simulink model "Grid_Forming_Converters_Microgrid_Github"  (R2020b)
settings: Solver=VariableStepAuto  StartTime=0.0  StopTime=1  RelTol=1e-3
values from neighbouring files (symbols this model uses):
  C_fi_1DG = 50*10^-6    (= 5e-05)    [Script_Primary_Secondary_Controller_GITHUB.m]
  C_fi_2DG = 50*10^-6    (= 5e-05)    [Script_Primary_Secondary_Controller_GITHUB.m]
  C_fi_3DG = 50*10^-6    (= 5e-05)    [Script_Primary_Secondary_Controller_GITHUB.m]
  C_fi_4DG = 50*10^-6    (= 5e-05)    [Script_Primary_Secondary_Controller_GITHUB.m]
  Kff_i_1DG = 0.75    [Script_Primary_Secondary_Controller_GITHUB.m]
  Kff_i_2DG = 0.75    [Script_Primary_Secondary_Controller_GITHUB.m]
  Kff_i_3DG = 0.75    [Script_Primary_Secondary_Controller_GITHUB.m]
  Kff_i_4DG = 0.75    [Script_Primary_Secondary_Controller_GITHUB.m]
  ki = 142500    [Script_Primary_Secondary_Controller_GITHUB.m]
  Kii_1DG = 20000    [Script_Primary_Secondary_Controller_GITHUB.m]
  Kii_2DG = 20000    [Script_Primary_Secondary_Controller_GITHUB.m]
  Kii_3DG = 16000    [Script_Primary_Secondary_Controller_GITHUB.m]
  Kii_4DG = 16000    [Script_Primary_Secondary_Controller_GITHUB.m]
  Kiv_1DG = 420    [Script_Primary_Secondary_Controller_GITHUB.m]
  Kiv_2DG = 420    [Script_Primary_Secondary_Controller_GITHUB.m]
  Kiv_3DG = 390    [Script_Primary_Secondary_Controller_GITHUB.m]
  Kiv_4DG = 390    [Script_Primary_Secondary_Controller_GITHUB.m]
  kp = 285    [Script_Primary_Secondary_Controller_GITHUB.m]
  Kpi_1DG = 15    [Script_Primary_Secondary_Controller_GITHUB.m]
  Kpi_2DG = 15    [Script_Primary_Secondary_Controller_GITHUB.m]
  Kpi_3DG = 10.5    [Script_Primary_Secondary_Controller_GITHUB.m]
  Kpi_4DG = 10.5    [Script_Primary_Secondary_Controller_GITHUB.m]
  Kpv_1DG = 0.1    [Script_Primary_Secondary_Controller_GITHUB.m]
  Kpv_2DG = 0.1    [Script_Primary_Secondary_Controller_GITHUB.m]
  Kpv_3DG = 0.05    [Script_Primary_Secondary_Controller_GITHUB.m]
  Kpv_4DG = 0.05    [Script_Primary_Secondary_Controller_GITHUB.m]
  L_ci_1DG = 0.35*10^-3    (= 0.00035)    [Script_Primary_Secondary_Controller_GITHUB.m]
  L_ci_2DG = 0.35*10^-3    (= 0.00035)    [Script_Primary_Secondary_Controller_GITHUB.m]
  L_fi_1DG = 1.35*10^-3    (= 0.00135)    [Script_Primary_Secondary_Controller_GITHUB.m]
  L_fi_2DG = 1.35*10^-3    (= 0.00135)    [Script_Primary_Secondary_Controller_GITHUB.m]
  L_fi_3DG = 1.35*10^-3    (= 0.00135)    [Script_Primary_Secondary_Controller_GITHUB.m]
  L_fi_4DG = 1.35*10^-3    (= 0.00135)    [Script_Primary_Secondary_Controller_GITHUB.m]
  L_line_1 = 318*10^-6    (= 0.000318)    [Script_Primary_Secondary_Controller_GITHUB.m]
  L_line_2 = 1847*10^-6    (= 0.001847)    [Script_Primary_Secondary_Controller_GITHUB.m]
  L_line_3 = 318*10^-6    (= 0.000318)    [Script_Primary_Secondary_Controller_GITHUB.m]
  L_load_1 = (X_load_1)/(2*pi*f)    (= 0.0477464829276)    [Script_Primary_Secondary_Controller_GITHUB.m]
  L_load_2 = (X_load_2)/(2*pi*f)    (= 0.0318309886184)    [Script_Primary_Secondary_Controller_GITHUB.m]
  L_load_3 = (X_load_3)/(2*pi*f)    (= 0.0318309886184)    [Script_Primary_Secondary_Controller_GITHUB.m]
  L_load_4 = (X_load_4)/(2*pi*f)    (= 0.0477464829276)    [Script_Primary_Secondary_Controller_GITHUB.m]
  m_P_1DG = 9.4*10^-5    (= 9.4e-05)    [Script_Primary_Secondary_Controller_GITHUB.m]
  m_P_2DG = 9.4*10^-5    (= 9.4e-05)    [Script_Primary_Secondary_Controller_GITHUB.m]
  m_P_3DG = 12.5*10^-5    (= 0.000125)    [Script_Primary_Secondary_Controller_GITHUB.m]
  m_P_4DG = 12.5*10^-5    (= 0.000125)    [Script_Primary_Secondary_Controller_GITHUB.m]
  n_Q_1DG = 1.3*10^-3    (= 0.0013)    [Script_Primary_Secondary_Controller_GITHUB.m]
  n_Q_2DG = 1.3*10^-3    (= 0.0013)    [Script_Primary_Secondary_Controller_GITHUB.m]
  n_Q_3DG = 1.5*10^-3    (= 0.0015)    [Script_Primary_Secondary_Controller_GITHUB.m]
  n_Q_4DG = 1.5*10^-3    (= 0.0015)    [Script_Primary_Secondary_Controller_GITHUB.m]
  R_ci_1DG = 0.03    [Script_Primary_Secondary_Controller_GITHUB.m]
  R_ci_2DG = 0.03    [Script_Primary_Secondary_Controller_GITHUB.m]
  R_fi_1DG = 0.1    [Script_Primary_Secondary_Controller_GITHUB.m]
  R_fi_2DG = 0.1    [Script_Primary_Secondary_Controller_GITHUB.m]
  R_fi_3DG = 0.1    [Script_Primary_Secondary_Controller_GITHUB.m]
  R_line_1 = 0.23    [Script_Primary_Secondary_Controller_GITHUB.m]
  R_line_2 = 0.35    [Script_Primary_Secondary_Controller_GITHUB.m]
  R_line_3 = 0.23    [Script_Primary_Secondary_Controller_GITHUB.m]
  R_load_1 = 30    [Script_Primary_Secondary_Controller_GITHUB.m]
  R_load_2 = 20    [Script_Primary_Secondary_Controller_GITHUB.m]
  R_load_3 = 25    [Script_Primary_Secondary_Controller_GITHUB.m]
  R_load_4 = 25    [Script_Primary_Secondary_Controller_GITHUB.m]
  Ts_1DG = 2e-6    (= 2e-06)    [Script_Primary_Secondary_Controller_GITHUB.m]
  w_base_1DG = 2*pi*f_1DG    (= 314.159265359)    [Script_Primary_Secondary_Controller_GITHUB.m]
  w_base_2DG = 2*pi*f_2DG    (= 314.159265359)    [Script_Primary_Secondary_Controller_GITHUB.m]
  w_base_3DG = 2*pi*f_3DG    (= 314.159265359)    [Script_Primary_Secondary_Controller_GITHUB.m]
  w_base_4DG = 2*pi*f_4DG    (= 314.159265359)    [Script_Primary_Secondary_Controller_GITHUB.m]
  wci_1DG = 31.41    [Script_Primary_Secondary_Controller_GITHUB.m]
  wci_2DG = 31.41    [Script_Primary_Secondary_Controller_GITHUB.m]
  wci_3DG = 31.41    [Script_Primary_Secondary_Controller_GITHUB.m]
  wci_4DG = 31.41    [Script_Primary_Secondary_Controller_GITHUB.m]
undefined symbols (not defined in the file or in its folder): L_i_1DG
libraries: powerlib x140, powerlib_meascontrol x68, pid_lib x20
(part 2 of 6)

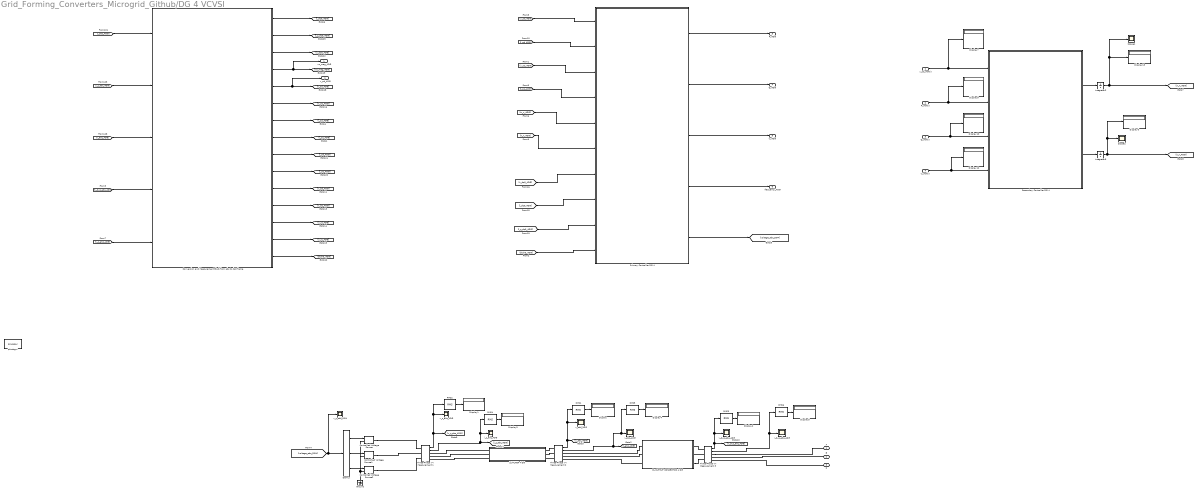
== system Grid_Forming_Converters_Microgrid_Github/DG 4 VCVSI  ==
  v_od_matrix : Inport
  P_matrix : Inport  Port=2
  Q_matrix : Inport  Port=3
  w_matrix : Inport  Port=4
  Controlled Voltage Source : powerlib/Electrical Sources/Controlled Voltage Source  Initialize=on  Source_Type=AC  Amplitude=0  Phase=0  Frequency=0  Measurements=None
  Controlled Voltage Source1 : powerlib/Electrical Sources/Controlled Voltage Source  Initialize=on  Source_Type=AC  Amplitude=0  Phase=0  Frequency=0  Measurements=None
  Controlled Voltage Source2 : powerlib/Electrical Sources/Controlled Voltage Source  Initialize=on  Source_Type=AC  Amplitude=0  Phase=0  Frequency=0  Measurements=None
  Conversion and Measurement Block from abc to dq0 frame : Subsystem
  Demux : Demux  Outputs=3
  Display{,1..7,9..10,12..13} (12 alike) : Display
  Ground : powerlib/Elements/Ground  LConnTagsString=a
  Integrator2 : Integrator
  Integrator3 : Integrator
  LC FILTER 4 DG : Subsystem
  Primary Controller DG 4 : Subsystem
  RL OUTPUT CONNECTOR 4 DG : Subsystem
  RMS{1..3,5..6} (5 alike) : powerlib_meascontrol/Measurements/RMS  TrueRMS=off  Freq=50  RMSInit=1  Ts=Ts_1DG
  RMS4 : powerlib_meascontrol/Measurements/RMS  TrueRMS=on  Freq=50  RMSInit=1  Ts=Ts_1DG
  Scope1 : Scope
  Scope2 : Scope
  Secondary Controller DG 4 : MATLAB Function  TreatAsAtomicUnit=on
  Three-Phase V-I Measurement 1 : powerlib/Measurements/Three-Phase V-I Measurement  VoltageMeasurement=phase-to-phase  SetLabelV=off  LabelV=Vabc  Vpu=off  VpuLL=off  CurrentMeasurement=yes  SetLabelI=off  LabelI=Iabc  Ipu=off  Pbase=45000  Vbase=380  OutputType=Complex  PhasorSimulation=off  PSBequivalent=0
  Three-Phase V-I Measurement 2 : powerlib/Measurements/Three-Phase V-I Measurement  VoltageMeasurement=phase-to-phase  SetLabelV=off  LabelV=Vabc  Vpu=off  VpuLL=off  CurrentMeasurement=yes  SetLabelI=off  LabelI=Iabc  Ipu=off  Pbase=45000  Vbase=380  OutputType=Complex  PhasorSimulation=off  PSBequivalent=0
  Three-Phase V-I Measurement 3 : powerlib/Measurements/Three-Phase V-I Measurement  VoltageMeasurement=phase-to-phase  SetLabelV=off  LabelV=Vabc  Vpu=off  VpuLL=off  CurrentMeasurement=yes  SetLabelI=off  LabelI=Iabc  Ipu=off  Pbase=45000  Vbase=380  OutputType=Complex  PhasorSimulation=off  PSBequivalent=0
  i_abc_4DG : Scope
  i_bus_abc_4DG : Scope
  i_s_abc_4DG : Scope
  powergui : powerlib/powergui  Priority=1  SimulationMode=Discrete  SampleTime=2e-6  frequency=60  Iterations=50  frequencyindice=0  Pbase=100e6  ErrMax=1e-4  UnitsV=kV  UnitsW=MW  buscounter=0  FunctionMessages=off  echomessages=off  EnableUseOfTLC=off  CurrentSourceSwitches=off  DisableSnubberDevices=off  DisableRonSwitches=off  DisableVfSwitches=off  DisplayEquations=off  AutomaticDiscreteSolvers=off  SolverType=Tustin/Backward Euler (TBE)  Interpol=off  ExternalGateDelay=off  methode=off  Ts=100  x0status=blocks  SPID=on  SwTol=0  HookPort=off  NonlinearTolerance=1e-4  nMaxIteration=100  ContinueOnMaxIteration=off  RestoreLinks=warning  ResistiveCurrentMeasurement=off  Frange=[0:2:500]  Ylog=off  Xlog=on  ShowGrid=off  save=off  variable=ZData  structure=0  ZoomFFT=off  StartTime=0.0  cycles=1  DisplayStyle=1  fundamental=60  FreqAxis=off  MaxFrequency=1000  frequencyindicesteady=1  RmsSteady=1  display=off
  v_abc_4DG : Scope
  v_bus_abc_4DG : Scope
  v_s_abc_4DG : Scope
  v_s_abc_DG4 : Scope
  A : PMIOPort  Side=Right
  B : PMIOPort  Port=2  Side=Right
  C : PMIOPort  Port=3  Side=Right
  vo_mag_4DG : Outport
  v_od_4DG : Outport  Port=2
  P_4DG : Outport  Port=3
  Q_4DG : Outport  Port=4
  w_4DG : Outport  Port=5
  frequency_4DG : Outport  Port=6
  wires:
  Three-Phase V-I Measurement 2/1 -> RMS1/1, v_abc_4DG/1, [v_abc_4DG]
  Three-Phase V-I Measurement 1/1 -> [v_s_abc_4DG], RMS2/1, v_s_abc_4DG/1
  Three-Phase V-I Measurement 1/2 -> RMS4/1, i_s_abc_4DG/1, [i_s_abc_4DG]
  RMS3/1 -> Display2/1
  Three-Phase V-I Measurement 3/1 -> [v_bus_abc_4DG], RMS3/1, v_bus_abc_4DG/1
  RMS5/1 -> Display4/1
  Three-Phase V-I Measurement 2/2 -> RMS5/1, i_abc_4DG/1, [i_abc_4DG]
  RMS1/1 -> Display/1
  Three-Phase V-I Measurement 3/2 -> RMS6/1, i_bus_abc_4DG/1
  RMS6/1 -> Display5/1
  RMS2/1 -> Display1/1
  RMS4/1 -> Display3/1
  Primary Controller DG 4/1(P_4DG) -> P_4DG/1
  Primary Controller DG 4/5(voltage_abc_DG4) -> [voltage_abc_DG4]
  [V_n_4DG] -> Primary Controller DG 4/6(V_n_4DG)
  Primary Controller DG 4/4(frequency_4DG) -> frequency_4DG/1
  [w_n_4DG] -> Primary Controller DG 4/5(w_n_4DG)
  [voltage_abc_DG4] -> Demux/1, v_s_abc_DG4/1
  Demux/1 -> Controlled Voltage Source/1
  Demux/2 -> Controlled Voltage Source1/1
  Demux/3 -> Controlled Voltage Source2/1
  [i_abc_4DG] -> Conversion and Measurement Block from abc to dq0 frame/1(i_abc_4DG)
  [i_s_abc_4DG] -> Conversion and Measurement Block from abc to dq0 frame/2(i_s_abc_4DG)
  [v_abc_4DG] -> Conversion and Measurement Block from abc to dq0 frame/3(v_abc_4DG)
  Conversion and Measurement Block from abc to dq0 frame/8(i_1q_4DG) -> [i_1q_4DG]
  Conversion and Measurement Block from abc to dq0 frame/7(i_1d_4DG) -> [i_1d_4DG]
  Conversion and Measurement Block from abc to dq0 frame/6(v_oq_4DG) -> [v_oq_4DG]
  Conversion and Measurement Block from abc to dq0 frame/4(vo_mag_4DG) -> [vo_mag_4DG], vo_mag_4DG/1
  Conversion and Measurement Block from abc to dq0 frame/5(v_od_4DG) -> [v_od_4DG], v_od_4DG/1
  [i_oq_4DG] -> Primary Controller DG 4/4(i_oq_4DG)
  [v_od_4DG] -> Primary Controller DG 4/1(v_od_4DG)
  [v_oq_4DG] -> Primary Controller DG 4/3(v_oq_4DG)
  [i_od_4DG] -> Primary Controller DG 4/2(i_od_4DG)
  [i_dq0_4DG] -> Primary Controller DG 4/8(i_dq0_4DG)
  [v_dq0_4DG] -> Primary Controller DG 4/7(v_dq0_4DG)
  [i_s_dq0_4DG] -> Primary Controller DG 4/9(i_s_dq0_4DG)
  Conversion and Measurement Block from abc to dq0 frame/9(i_od_4DG) -> [i_od_4DG]
  Conversion and Measurement Block from abc to dq0 frame/10(i_oq_4DG) -> [i_oq_4DG]
  Conversion and Measurement Block from abc to dq0 frame/15(alpha_4DG) -> [alpha_4DG]
  Conversion and Measurement Block from abc to dq0 frame/1(i_dq0_4DG) -> [i_dq0_4DG]
  Conversion and Measurement Block from abc to dq0 frame/2(i_s_dq0_4DG) -> [i_s_dq0_4DG]
  Conversion and Measurement Block from abc to dq0 frame/3(v_dq0_4DG) -> [v_dq0_4DG]
  [alpha_4DG] -> Primary Controller DG 4/10(alpha_4DG)
  Primary Controller DG 4/3(w_4DG) -> w_4DG/1
  Primary Controller DG 4/2(Q_4DG) -> Q_4DG/1
  [v_bus_abc_4DG] -> Conversion and Measurement Block from abc to dq0 frame/4(v_bus_abc_4DG)
  [v_s_abc_4DG] -> Conversion and Measurement Block from abc to dq0 frame/5(v_s_abc_4DG)
  Conversion and Measurement Block from abc to dq0 frame/11(v_bd_4DG) -> [v_bd_4DG]
  Conversion and Measurement Block from abc to dq0 frame/12(v_bq_4DG) -> [v_bq_4DG]
  Conversion and Measurement Block from abc to dq0 frame/14(v_iq_4DG) -> [v_iq_4DG]
  Conversion and Measurement Block from abc to dq0 frame/13(v_id_4DG) -> [v_id_4DG]
  Integrator3/1 -> [V_n_4DG], Display6/1, Scope2/1
  Secondary Controller DG 4/1(v_f_4DG) -> Integrator2/1
  Integrator2/1 -> [w_n_4DG], Scope1/1, Display13/1
  Secondary Controller DG 4/2(v_v_4DG) -> Integrator3/1
  v_od_matrix/1 -> Display7/1, Secondary Controller DG 4/1(v_od_matrix)
  P_matrix/1 -> Display9/1, Secondary Controller DG 4/2(P_matrix)
  Q_matrix/1 -> Display10/1, Secondary Controller DG 4/3(Q_matrix)
  w_matrix/1 -> Display12/1, Secondary Controller DG 4/4(w_matrix)
  connections:
  RL OUTPUT CONNECTOR 4 DG/LConn2 -- Three-Phase V-I Measurement 2/RConn2
  LC FILTER 4 DG/LConn2 -- Three-Phase V-I Measurement 1/RConn2
  RL OUTPUT CONNECTOR 4 DG/LConn1 -- Three-Phase V-I Measurement 2/RConn1
  C/RConn1 -- Three-Phase V-I Measurement 3/RConn3
  Three-Phase V-I Measurement 2/LConn3 -- LC FILTER 4 DG/RConn3
  Three-Phase V-I Measurement 3/RConn1 -- A/RConn1
  B/RConn1 -- Three-Phase V-I Measurement 3/RConn2
  Controlled Voltage Source1/RConn1 -- Three-Phase V-I Measurement 1/LConn2
  RL OUTPUT CONNECTOR 4 DG/LConn3 -- Three-Phase V-I Measurement 2/RConn3
  Three-Phase V-I Measurement 3/LConn1 -- RL OUTPUT CONNECTOR 4 DG/RConn1
  Three-Phase V-I Measurement 2/LConn1 -- LC FILTER 4 DG/RConn1
  Three-Phase V-I Measurement 3/LConn2 -- RL OUTPUT CONNECTOR 4 DG/RConn2
  RL OUTPUT CONNECTOR 4 DG/RConn3 -- Three-Phase V-I Measurement 3/LConn3
  Controlled Voltage Source2/RConn1 -- Three-Phase V-I Measurement 1/LConn3
  LC FILTER 4 DG/LConn3 -- Three-Phase V-I Measurement 1/RConn3
  LC FILTER 4 DG/LConn1 -- Three-Phase V-I Measurement 1/RConn1
  Three-Phase V-I Measurement 2/LConn2 -- LC FILTER 4 DG/RConn2
  Controlled Voltage Source/RConn1 -- Three-Phase V-I Measurement 1/LConn1
  Ground/LConn1 -- Controlled Voltage Source/LConn1 -- Controlled Voltage Source1/LConn1 -- Controlled Voltage Source2/LConn1

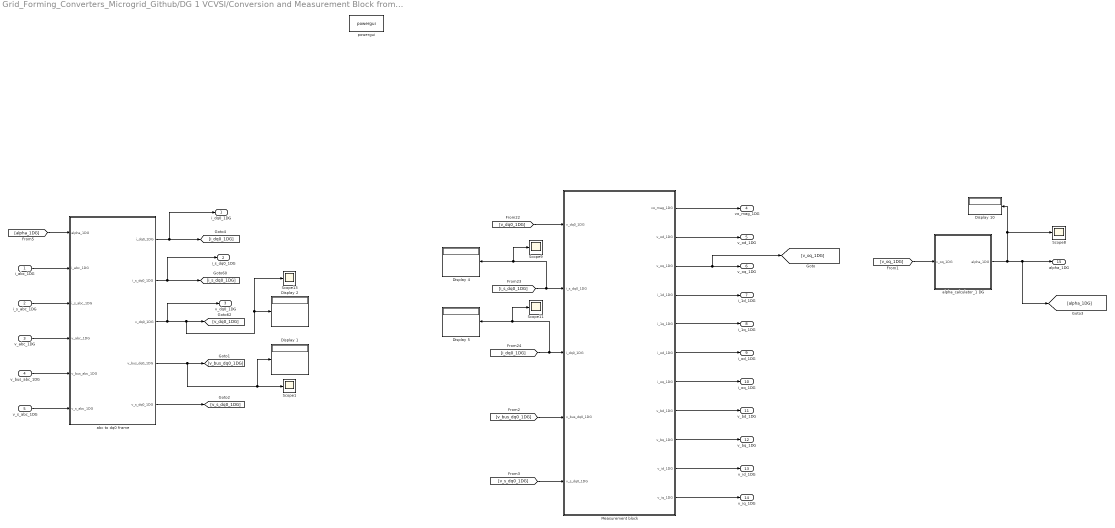
== system Grid_Forming_Converters_Microgrid_Github/DG 1 VCVSI/Conversion and Measurement Block from abc to dq0 frame ==
  i_abc_1DG : Inport
  i_s_abc_1DG : Inport  Port=2
  v_abc_1DG : Inport  Port=3
  v_bus_abc_1DG : Inport  Port=4
  v_s_abc_1DG : Inport  Port=5
  Display {1..2,4..5,10} (5 alike) : Display
      settings: Format=bank
  Measurement block : Subsystem
  Scope{1,8..9,11,13} (5 alike) : Scope
  abc to dq0 frame : Subsystem
  alpha_calculator_1 DG : Subsystem
  powergui : powerlib/powergui  Priority=1  SimulationMode=Discrete  SampleTime=2e-6  frequency=60  Iterations=50  frequencyindice=0  Pbase=100e6  ErrMax=1e-4  UnitsV=kV  UnitsW=MW  buscounter=0  FunctionMessages=off  echomessages=off  EnableUseOfTLC=off  CurrentSourceSwitches=off  DisableSnubberDevices=off  DisableRonSwitches=off  DisableVfSwitches=off  DisplayEquations=off  AutomaticDiscreteSolvers=off  SolverType=Tustin/Backward Euler (TBE)  Interpol=off  ExternalGateDelay=off  methode=off  Ts=100  x0status=blocks  SPID=on  SwTol=0  HookPort=off  NonlinearTolerance=1e-4  nMaxIteration=100  ContinueOnMaxIteration=off  RestoreLinks=warning  ResistiveCurrentMeasurement=off  Frange=[0:2:500]  Ylog=off  Xlog=on  ShowGrid=off  save=off  variable=ZData  structure=0  ZoomFFT=off  StartTime=0.0  cycles=1  DisplayStyle=1  fundamental=60  FreqAxis=off  MaxFrequency=1000  frequencyindicesteady=1  RmsSteady=1  display=off
  i_dq0_1DG : Outport
  i_s_dq0_1DG : Outport  Port=2
  v_dq0_1DG : Outport  Port=3
  vo_mag_1DG : Outport  Port=4
  v_od_1DG : Outport  Port=5
  v_oq_1DG : Outport  Port=6
  i_1d_1DG : Outport  Port=7
  i_1q_1DG : Outport  Port=8
  i_od_1DG : Outport  Port=9
  i_oq_1DG : Outport  Port=10
  v_bd_1DG : Outport  Port=11
  v_bq_1DG : Outport  Port=12
  v_id_1DG : Outport  Port=13
  v_iq_1DG : Outport  Port=14
  alpha_1DG : Outport  Port=15
  wires:
  Measurement block/5(i_1q_1DG) -> i_1q_1DG/1
  [i_dq0_1DG] -> Scope11/1, Display 5/1, Measurement block/3(i_dq0_1DG)
  abc to dq0 frame/2(i_s_dq0_1DG) -> i_s_dq0_1DG/1, [i_s_dq0_1DG]
  i_s_abc_1DG/1 -> abc to dq0 frame/3(i_s_abc_1DG)
  abc to dq0 frame/1(i_dq0_1DG) -> i_dq0_1DG/1, [i_dq0_1DG]
  Measurement block/4(i_1d_1DG) -> i_1d_1DG/1
  Measurement block/6(i_od_1DG) -> i_od_1DG/1
  abc to dq0 frame/3(v_dq0_1DG) -> v_dq0_1DG/1, Scope13/1, Display 2/1, [v_dq0_1DG]
  [v_dq0_1DG] -> Measurement block/1(v_dq0_1DG)
  i_abc_1DG/1 -> abc to dq0 frame/2(i_abc_1DG)
  Measurement block/2(v_od_1DG) -> v_od_1DG/1
  Measurement block/3(v_oq_1DG) -> [v_oq_1DG], v_oq_1DG/1
  v_abc_1DG/1 -> abc to dq0 frame/4(v_abc_1DG)
  Measurement block/7(i_oq_1DG) -> i_oq_1DG/1
  alpha_calculator_1 DG/1(alpha_1DG) -> [alpha_1DG], alpha_1DG/1, Display 10/1, Scope8/1
  [v_oq_1DG] -> alpha_calculator_1 DG/1(v_oq_1DG)
  [alpha_1DG] -> abc to dq0 frame/1(alpha_1DG)
  Measurement block/1(vo_mag_1DG) -> vo_mag_1DG/1
  [i_s_dq0_1DG] -> Scope9/1, Display 4/1, Measurement block/2(i_s_dq0_1DG)
  abc to dq0 frame/4(v_bus_dq0_1DG) -> [v_bus_dq0_1DG], Scope1/1, Display 1/1
  v_bus_abc_1DG/1 -> abc to dq0 frame/5(v_bus_abc_1DG)
  [v_bus_dq0_1DG] -> Measurement block/4(v_bus_dq0_1DG)
  Measurement block/8(v_bd_1DG) -> v_bd_1DG/1
  Measurement block/9(v_bq_1DG) -> v_bq_1DG/1
  v_s_abc_1DG/1 -> abc to dq0 frame/6(v_s_abc_1DG)
  abc to dq0 frame/5(v_s_dq0_1DG) -> [v_s_dq0_1DG]
  [v_s_dq0_1DG] -> Measurement block/5(v_s_dq0_1DG)
  Measurement block/10(v_id_1DG) -> v_id_1DG/1
  Measurement block/11(v_iq_1DG) -> v_iq_1DG/1

== system Grid_Forming_Converters_Microgrid_Github/DG 1 VCVSI/LC FILTER 1 DG ==
  C_a : powerlib/Elements/Series RLC Branch  LConnTagsString=__new0  RConnTagsString=__new0  BranchType=C  Resistance=1  Inductance=1e-3  SetiL0=off  InitialCurrent=0  Capacitance=C_fi_1DG  Setx0=off  InitialVoltage=165  Measurements=None
  C_b : powerlib/Elements/Series RLC Branch  LConnTagsString=__new0  RConnTagsString=__new0  BranchType=C  Resistance=1  Inductance=1e-3  SetiL0=off  InitialCurrent=0  Capacitance=C_fi_1DG  Setx0=off  InitialVoltage=165  Measurements=None
  C_c1 : powerlib/Elements/Series RLC Branch  LConnTagsString=__new0  RConnTagsString=__new0  BranchType=C  Resistance=1  Inductance=1e-3  SetiL0=off  InitialCurrent=0  Capacitance=C_fi_1DG  Setx0=off  InitialVoltage=165  Measurements=None
  Ground2 : powerlib/Elements/Ground  LConnTagsString=a
  Series RLC Branch : powerlib/Elements/Series RLC Branch  LConnTagsString=__new0  RConnTagsString=__new0  BranchType=L  Resistance=1  Inductance=L_fi_1DG  SetiL0=off  InitialCurrent=0  Capacitance=1e-6  Setx0=off  InitialVoltage=0  Measurements=None
  Series RLC Branch1 : powerlib/Elements/Series RLC Branch  LConnTagsString=__new0  RConnTagsString=__new0  BranchType=R  Resistance=R_fi_1DG  Inductance=L_i_1DG  SetiL0=off  InitialCurrent=0  Capacitance=1e-6  Setx0=off  InitialVoltage=0  Measurements=None
  Series RLC Branch2 : powerlib/Elements/Series RLC Branch  LConnTagsString=__new0  RConnTagsString=__new0  BranchType=R  Resistance=R_fi_1DG  Inductance=L_i_1DG  SetiL0=off  InitialCurrent=0  Capacitance=1e-6  Setx0=off  InitialVoltage=0  Measurements=None
  Series RLC Branch3 : powerlib/Elements/Series RLC Branch  LConnTagsString=__new0  RConnTagsString=__new0  BranchType=L  Resistance=1  Inductance=L_fi_1DG  SetiL0=off  InitialCurrent=0  Capacitance=1e-6  Setx0=off  InitialVoltage=0  Measurements=None
  Series RLC Branch4 : powerlib/Elements/Series RLC Branch  LConnTagsString=__new0  RConnTagsString=__new0  BranchType=R  Resistance=R_fi_1DG  Inductance=R_fi_1DG  SetiL0=off  InitialCurrent=0  Capacitance=1e-6  Setx0=off  InitialVoltage=0  Measurements=None
  Series RLC Branch5 : powerlib/Elements/Series RLC Branch  LConnTagsString=__new0  RConnTagsString=__new0  BranchType=L  Resistance=1  Inductance=L_fi_1DG  SetiL0=off  InitialCurrent=0  Capacitance=1e-6  Setx0=off  InitialVoltage=0  Measurements=None
  Series RLC Branch6 : PMIOPort  Side=Left
  Series RLC Branch7 : PMIOPort  Port=2  Side=Right
  Series RLC Branch8 : PMIOPort  Port=3  Side=Left
  Series RLC Branch9 : PMIOPort  Port=4  Side=Right
  Series RLC Branch10 : PMIOPort  Port=5  Side=Left
  Series RLC Branch11 : PMIOPort  Port=6  Side=Right
  connections:
  Series RLC Branch7/RConn1 -- C_c1/LConn1 -- Series RLC Branch/RConn1
  Series RLC Branch8/RConn1 -- Series RLC Branch2/LConn1
  Series RLC Branch6/RConn1 -- Series RLC Branch1/LConn1
  Series RLC Branch9/RConn1 -- C_b/LConn1 -- Series RLC Branch3/RConn1
  Series RLC Branch11/RConn1 -- C_a/LConn1 -- Series RLC Branch5/RConn1
  Series RLC Branch10/RConn1 -- Series RLC Branch4/LConn1
  C_b/RConn1 -- C_c1/RConn1 -- Ground2/LConn1 -- C_a/RConn1
  Series RLC Branch/LConn1 -- Series RLC Branch1/RConn1
  Series RLC Branch3/LConn1 -- Series RLC Branch2/RConn1
  Series RLC Branch4/RConn1 -- Series RLC Branch5/LConn1

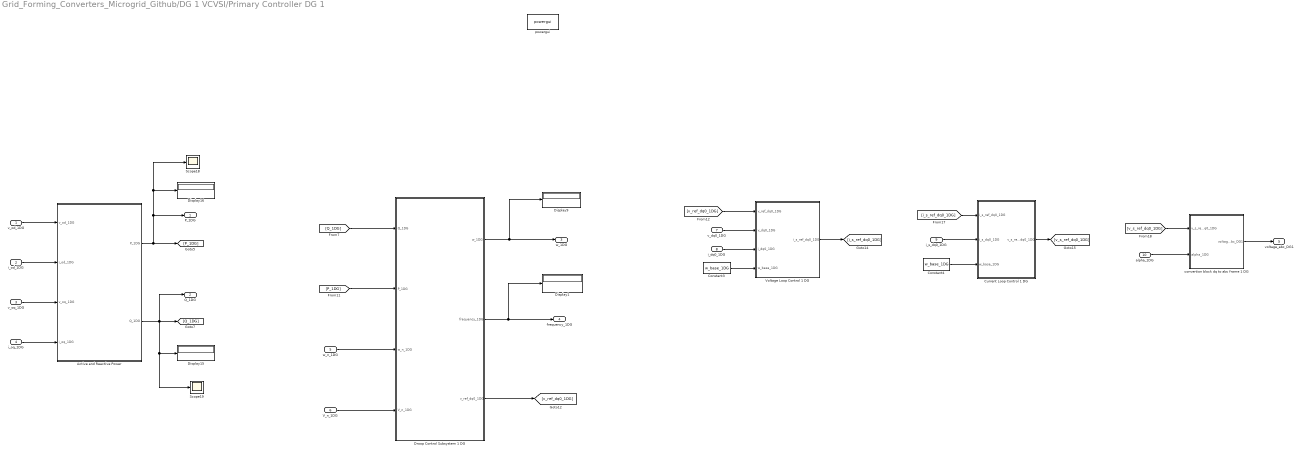
== system Grid_Forming_Converters_Microgrid_Github/DG 1 VCVSI/Primary Controller DG 1 ==
  v_od_1DG : Inport
  i_od_1DG : Inport  Port=2
  v_oq_1DG : Inport  Port=3
  i_oq_1DG : Inport  Port=4
  w_n_1DG : Inport  Port=5
  V_n_1DG : Inport  Port=6
  v_dq0_1DG : Inport  Port=7
  i_dq0_1DG : Inport  Port=8
  i_s_dq0_1DG : Inport  Port=9
  alpha_1DG : Inport  Port=10
  Active and Reactive Power : Subsystem
  Constant3 : Constant  Value=w_base_1DG
  Constant4 : Constant  Value=w_base_1DG
  Current Loop Control 1 DG : Subsystem
  Display{1,9,15..16} (4 alike) : Display
  Droop Control Subsystem 1 DG : Subsystem
  Scope18 : Scope
  Scope19 : Scope
  Voltage Loop Control 1 DG : Subsystem
  convertion block dq to abc frame 1 DG : Subsystem
  powergui : powerlib/powergui  Priority=1  SimulationMode=Discrete  SampleTime=Ts_1DG  frequency=60  Iterations=50  frequencyindice=0  Pbase=100e6  ErrMax=1e-4  UnitsV=kV  UnitsW=MW  buscounter=0  FunctionMessages=off  echomessages=off  EnableUseOfTLC=off  CurrentSourceSwitches=off  DisableSnubberDevices=off  DisableRonSwitches=off  DisableVfSwitches=off  DisplayEquations=off  AutomaticDiscreteSolvers=off  SolverType=Tustin/Backward Euler (TBE)  Interpol=off  ExternalGateDelay=off  methode=off  Ts=100  x0status=blocks  SPID=on  SwTol=0  HookPort=off  NonlinearTolerance=1e-4  nMaxIteration=100  ContinueOnMaxIteration=off  RestoreLinks=warning  ResistiveCurrentMeasurement=off  Frange=[0:2:500]  Ylog=off  Xlog=on  ShowGrid=off  save=off  variable=ZData  structure=0  ZoomFFT=off  StartTime=0.0  cycles=1  DisplayStyle=1  fundamental=60  FreqAxis=off  MaxFrequency=1000  frequencyindicesteady=1  RmsSteady=1  display=off
  P_1DG : Outport
  Q_1DG : Outport  Port=2
  w_1DG : Outport  Port=3
  frequency_1DG : Outport  Port=4
  voltage_abc_DG1 : Outport  Port=5
  wires:
  Active and Reactive Power/2(Q_1DG) -> Display15/1, Scope19/1, Q_1DG/1, [Q_1DG]
  Voltage Loop Control 1 DG/1(i_s_ref_dq0_1DG) -> [i_s_ref_dq0_1DG]
  Active and Reactive Power/1(P_1DG) -> P_1DG/1, Scope18/1, Display16/1, [P_1DG]
  [v_ref_dq0_1DG] -> Voltage Loop Control 1 DG/1(v_ref_dq0_1DG)
  [P_1DG] -> Droop Control Subsystem 1 DG/2(P_1DG)
  Current Loop Control 1 DG/1(v_s_ref_dq0_1DG) -> [v_s_ref_dq0_1DG]
  Constant4/1 -> Current Loop Control 1 DG/3(w_base_1DG)
  v_dq0_1DG/1 -> Voltage Loop Control 1 DG/2(v_dq0_1DG)
  Droop Control Subsystem 1 DG/3(v_ref_dq0_1DG) -> [v_ref_dq0_1DG]
  [Q_1DG] -> Droop Control Subsystem 1 DG/1(Q_1DG)
  Droop Control Subsystem 1 DG/1(w_1DG) -> Display9/1, w_1DG/1
  i_dq0_1DG/1 -> Voltage Loop Control 1 DG/3(i_dq0_1DG)
  i_s_dq0_1DG/1 -> Current Loop Control 1 DG/2(i_s_dq0_1DG)
  Constant3/1 -> Voltage Loop Control 1 DG/4(w_base_1DG)
  [i_s_ref_dq0_1DG] -> Current Loop Control 1 DG/1(i_s_ref_dq0_1DG)
  convertion block dq to abc frame 1 DG/1(voltage_abc_DG1) -> voltage_abc_DG1/1
  [v_s_ref_dq0_1DG] -> convertion block dq to abc frame 1 DG/1(v_s_ref_dq0_1DG)
  alpha_1DG/1 -> convertion block dq to abc frame 1 DG/2(alpha_1DG)
  V_n_1DG/1 -> Droop Control Subsystem 1 DG/4(V_n_1DG)
  v_od_1DG/1 -> Active and Reactive Power/1(v_od_1DG)
  i_oq_1DG/1 -> Active and Reactive Power/4(i_oq_1DG)
  v_oq_1DG/1 -> Active and Reactive Power/3(v_oq_1DG)
  i_od_1DG/1 -> Active and Reactive Power/2(i_od_1DG)
  w_n_1DG/1 -> Droop Control Subsystem 1 DG/3(w_n_1DG)
  Droop Control Subsystem 1 DG/2(frequency_1DG) -> Display1/1, frequency_1DG/1

== system Grid_Forming_Converters_Microgrid_Github/DG 1 VCVSI/RL OUTPUT CONNECTOR 1 DG ==
  Series RLC Branch : powerlib/Elements/Series RLC Branch  LConnTagsString=__new0  RConnTagsString=__new0  BranchType=RL  Resistance=R_ci_1DG  Inductance=L_ci_1DG  SetiL0=off  InitialCurrent=0  Capacitance=1e-6  Setx0=off  InitialVoltage=0  Measurements=None
  Series RLC Branch1 : powerlib/Elements/Series RLC Branch  LConnTagsString=__new0  RConnTagsString=__new0  BranchType=RL  Resistance=R_ci_1DG  Inductance=L_ci_1DG  SetiL0=off  InitialCurrent=0  Capacitance=1e-6  Setx0=off  InitialVoltage=0  Measurements=None
  Series RLC Branch2 : powerlib/Elements/Series RLC Branch  LConnTagsString=__new0  RConnTagsString=__new0  BranchType=RL  Resistance=R_ci_1DG  Inductance=L_ci_1DG  SetiL0=off  InitialCurrent=0  Capacitance=1e-6  Setx0=off  InitialVoltage=0  Measurements=None
  Series RLC Branch3 : PMIOPort  Side=Right
  Series RLC Branch4 : PMIOPort  Port=2  Side=Left
  Series RLC Branch5 : PMIOPort  Port=3  Side=Right
  Series RLC Branch6 : PMIOPort  Port=4  Side=Left
  Series RLC Branch7 : PMIOPort  Port=5  Side=Left
  Series RLC Branch8 : PMIOPort  Port=6  Side=Right
  connections:
  Series RLC Branch1/LConn1 -- Series RLC Branch6/RConn1
  Series RLC Branch2/RConn1 -- Series RLC Branch8/RConn1
  Series RLC Branch/RConn1 -- Series RLC Branch3/RConn1
  Series RLC Branch2/LConn1 -- Series RLC Branch7/RConn1
  Series RLC Branch/LConn1 -- Series RLC Branch4/RConn1
  Series RLC Branch1/RConn1 -- Series RLC Branch5/RConn1

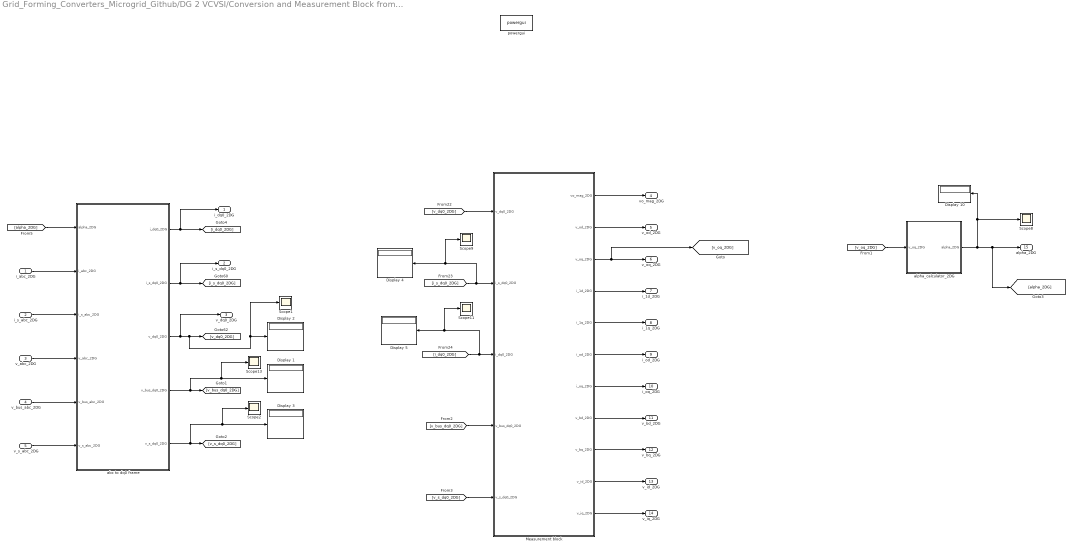
== system Grid_Forming_Converters_Microgrid_Github/DG 2 VCVSI/Conversion and Measurement Block from abc to dq0 frame ==
  i_abc_2DG : Inport
  i_s_abc_2DG : Inport  Port=2
  v_abc_2DG : Inport  Port=3
  v_bus_abc_2DG : Inport  Port=4
  v_s_abc_2DG : Inport  Port=5
  Display {1..5,10} (6 alike) : Display
      settings: Format=bank
  Measurement block : Subsystem
  Scope{1..2,8..9,11,13} (6 alike) : Scope
  abc to dq0 frame : Subsystem
  alpha_calculator_2DG : Subsystem
  powergui : powerlib/powergui  Priority=1  SimulationMode=Discrete  SampleTime=2e-6  frequency=60  Iterations=50  frequencyindice=0  Pbase=100e6  ErrMax=1e-4  UnitsV=kV  UnitsW=MW  buscounter=0  FunctionMessages=off  echomessages=off  EnableUseOfTLC=off  CurrentSourceSwitches=off  DisableSnubberDevices=off  DisableRonSwitches=off  DisableVfSwitches=off  DisplayEquations=off  AutomaticDiscreteSolvers=off  SolverType=Tustin/Backward Euler (TBE)  Interpol=off  ExternalGateDelay=off  methode=off  Ts=100  x0status=blocks  SPID=on  SwTol=0  HookPort=off  NonlinearTolerance=1e-4  nMaxIteration=100  ContinueOnMaxIteration=off  RestoreLinks=warning  ResistiveCurrentMeasurement=off  Frange=[0:2:500]  Ylog=off  Xlog=on  ShowGrid=off  save=off  variable=ZData  structure=0  ZoomFFT=off  StartTime=0.0  cycles=1  DisplayStyle=1  fundamental=60  FreqAxis=off  MaxFrequency=1000  frequencyindicesteady=1  RmsSteady=1  display=off
  i_dq0_2DG : Outport
  i_s_dq0_2DG : Outport  Port=2
  v_dq0_2DG : Outport  Port=3
  vo_mag_2DG : Outport  Port=4
  v_od_2DG : Outport  Port=5
  v_oq_2DG : Outport  Port=6
  i_1d_2DG : Outport  Port=7
  i_1q_2DG : Outport  Port=8
  i_od_2DG : Outport  Port=9
  i_oq_2DG : Outport  Port=10
  v_bd_2DG : Outport  Port=11
  v_bq_2DG : Outport  Port=12
  v_id_2DG : Outport  Port=13
  v_iq_2DG : Outport  Port=14
  alpha_2DG : Outport  Port=15
  wires:
  Measurement block/5(i_1q_2DG) -> i_1q_2DG/1
  [i_dq0_2DG] -> Scope11/1, Display 5/1, Measurement block/3(i_dq0_2DG)
  abc to dq0 frame/2(i_s_dq0_2DG) -> i_s_dq0_2DG/1, [i_s_dq0_2DG]
  i_s_abc_2DG/1 -> abc to dq0 frame/3(i_s_abc_2DG)
  abc to dq0 frame/1(i_dq0_2DG) -> i_dq0_2DG/1, [i_dq0_2DG]
  Measurement block/4(i_1d_2DG) -> i_1d_2DG/1
  Measurement block/6(i_od_2DG) -> i_od_2DG/1
  abc to dq0 frame/3(v_dq0_2DG) -> v_dq0_2DG/1, Scope1/1, Display 2/1, [v_dq0_2DG]
  [v_dq0_2DG] -> Measurement block/1(v_dq0_2DG)
  i_abc_2DG/1 -> abc to dq0 frame/2(i_abc_2DG)
  Measurement block/2(v_od_2DG) -> v_od_2DG/1
  Measurement block/3(v_oq_2DG) -> [v_oq_2DG], v_oq_2DG/1
  v_abc_2DG/1 -> abc to dq0 frame/4(v_abc_2DG)
  Measurement block/7(i_oq_2DG) -> i_oq_2DG/1
  alpha_calculator_2DG/1(alpha_2DG) -> [alpha_2DG], alpha_2DG/1, Display 10/1, Scope8/1
  [v_oq_2DG] -> alpha_calculator_2DG/1(v_oq_2DG)
  [alpha_2DG] -> abc to dq0 frame/1(alpha_2DG)
  Measurement block/1(vo_mag_2DG) -> vo_mag_2DG/1
  [i_s_dq0_2DG] -> Scope9/1, Display 4/1, Measurement block/2(i_s_dq0_2DG)
  v_bus_abc_2DG/1 -> abc to dq0 frame/5(v_bus_abc_2DG)
  v_s_abc_2DG/1 -> abc to dq0 frame/6(v_s_abc_2DG)
  abc to dq0 frame/4(v_bus_dq0_2DG) -> Scope13/1, Display 1/1, [v_bus_dq0_2DG]
  abc to dq0 frame/5(v_s_dq0_2DG) -> Scope2/1, Display 3/1, [v_s_dq0_2DG]
  [v_bus_dq0_2DG] -> Measurement block/4(v_bus_dq0_2DG)
  [v_s_dq0_2DG] -> Measurement block/5(v_s_dq0_2DG)
  Measurement block/8(v_bd_2DG) -> v_bd_2DG/1
  Measurement block/9(v_bq_2DG) -> v_bq_2DG/1
  Measurement block/10(v_id_2DG) -> v_id_2DG/1
  Measurement block/11(v_iq_2DG) -> v_iq_2DG/1

== system Grid_Forming_Converters_Microgrid_Github/DG 2 VCVSI/LC FILTER 2 DG ==
  C_a : powerlib/Elements/Series RLC Branch  LConnTagsString=__new0  RConnTagsString=__new0  BranchType=C  Resistance=1  Inductance=1e-3  SetiL0=off  InitialCurrent=0  Capacitance=C_fi_2DG  Setx0=off  InitialVoltage=165  Measurements=None
  C_b : powerlib/Elements/Series RLC Branch  LConnTagsString=__new0  RConnTagsString=__new0  BranchType=C  Resistance=1  Inductance=1e-3  SetiL0=off  InitialCurrent=0  Capacitance=C_fi_2DG  Setx0=off  InitialVoltage=165  Measurements=None
  C_c1 : powerlib/Elements/Series RLC Branch  LConnTagsString=__new0  RConnTagsString=__new0  BranchType=C  Resistance=1  Inductance=1e-3  SetiL0=off  InitialCurrent=0  Capacitance=C_fi_2DG  Setx0=off  InitialVoltage=165  Measurements=None
  Ground2 : powerlib/Elements/Ground  LConnTagsString=a
  Series RLC Branch : powerlib/Elements/Series RLC Branch  LConnTagsString=__new0  RConnTagsString=__new0  BranchType=L  Resistance=1  Inductance=L_fi_2DG  SetiL0=off  InitialCurrent=0  Capacitance=1e-6  Setx0=off  InitialVoltage=0  Measurements=None
  Series RLC Branch1 : powerlib/Elements/Series RLC Branch  LConnTagsString=__new0  RConnTagsString=__new0  BranchType=R  Resistance=R_fi_2DG  Inductance=L_i_1DG  SetiL0=off  InitialCurrent=0  Capacitance=1e-6  Setx0=off  InitialVoltage=0  Measurements=None
  Series RLC Branch2 : powerlib/Elements/Series RLC Branch  LConnTagsString=__new0  RConnTagsString=__new0  BranchType=R  Resistance=R_fi_2DG  Inductance=L_i_1DG  SetiL0=off  InitialCurrent=0  Capacitance=1e-6  Setx0=off  InitialVoltage=0  Measurements=None
  Series RLC Branch3 : powerlib/Elements/Series RLC Branch  LConnTagsString=__new0  RConnTagsString=__new0  BranchType=L  Resistance=1  Inductance=L_fi_2DG  SetiL0=off  InitialCurrent=0  Capacitance=1e-6  Setx0=off  InitialVoltage=0  Measurements=None
  Series RLC Branch4 : powerlib/Elements/Series RLC Branch  LConnTagsString=__new0  RConnTagsString=__new0  BranchType=R  Resistance=R_fi_2DG  Inductance=R_fi_1DG  SetiL0=off  InitialCurrent=0  Capacitance=1e-6  Setx0=off  InitialVoltage=0  Measurements=None
  Series RLC Branch5 : powerlib/Elements/Series RLC Branch  LConnTagsString=__new0  RConnTagsString=__new0  BranchType=L  Resistance=1  Inductance=L_fi_2DG  SetiL0=off  InitialCurrent=0  Capacitance=1e-6  Setx0=off  InitialVoltage=0  Measurements=None
  Series RLC Branch6 : PMIOPort  Side=Left
  Series RLC Branch7 : PMIOPort  Port=2  Side=Right
  Series RLC Branch8 : PMIOPort  Port=3  Side=Left
  Series RLC Branch9 : PMIOPort  Port=4  Side=Right
  Series RLC Branch10 : PMIOPort  Port=5  Side=Left
  Series RLC Branch11 : PMIOPort  Port=6  Side=Right
  connections:
  Series RLC Branch7/RConn1 -- C_c1/LConn1 -- Series RLC Branch/RConn1
  Series RLC Branch8/RConn1 -- Series RLC Branch2/LConn1
  Series RLC Branch6/RConn1 -- Series RLC Branch1/LConn1
  Series RLC Branch9/RConn1 -- C_b/LConn1 -- Series RLC Branch3/RConn1
  Series RLC Branch11/RConn1 -- C_a/LConn1 -- Series RLC Branch5/RConn1
  Series RLC Branch10/RConn1 -- Series RLC Branch4/LConn1
  C_b/RConn1 -- C_c1/RConn1 -- Ground2/LConn1 -- C_a/RConn1
  Series RLC Branch/LConn1 -- Series RLC Branch1/RConn1
  Series RLC Branch3/LConn1 -- Series RLC Branch2/RConn1
  Series RLC Branch4/RConn1 -- Series RLC Branch5/LConn1

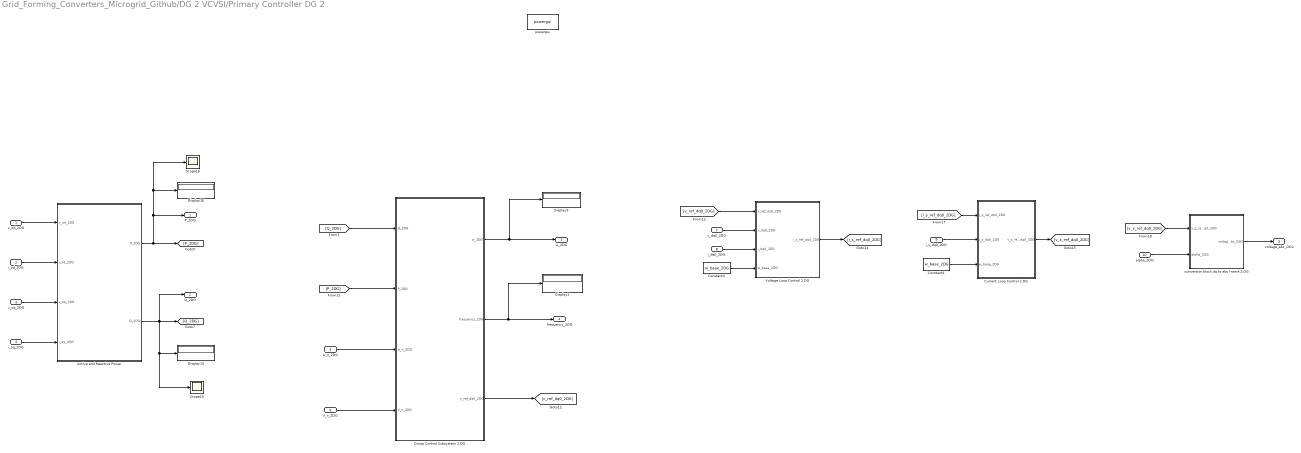
== system Grid_Forming_Converters_Microgrid_Github/DG 2 VCVSI/Primary Controller DG 2 ==
  v_od_2DG : Inport
  i_od_2DG : Inport  Port=2
  v_oq_2DG : Inport  Port=3
  i_oq_2DG : Inport  Port=4
  w_n_2DG : Inport  Port=5
  V_n_2DG : Inport  Port=6
  v_dq0_2DG : Inport  Port=7
  i_dq0_2DG : Inport  Port=8
  i_s_dq0_2DG : Inport  Port=9
  alpha_2DG : Inport  Port=10
  Active and Reactive Power : Subsystem
  Constant3 : Constant  Value=w_base_2DG
  Constant4 : Constant  Value=w_base_2DG
  Current Loop Control 2 DG : Subsystem
  Display{1,9,15..16} (4 alike) : Display
  Droop Control Subsystem 2 DG : Subsystem
  Scope18 : Scope
  Scope19 : Scope
  Voltage Loop Control 2 DG : Subsystem
  convertion block dq to abc frame 2 DG : Subsystem
  powergui : powerlib/powergui  Priority=1  SimulationMode=Discrete  SampleTime=Ts_1DG  frequency=60  Iterations=50  frequencyindice=0  Pbase=100e6  ErrMax=1e-4  UnitsV=kV  UnitsW=MW  buscounter=0  FunctionMessages=off  echomessages=off  EnableUseOfTLC=off  CurrentSourceSwitches=off  DisableSnubberDevices=off  DisableRonSwitches=off  DisableVfSwitches=off  DisplayEquations=off  AutomaticDiscreteSolvers=off  SolverType=Tustin/Backward Euler (TBE)  Interpol=off  ExternalGateDelay=off  methode=off  Ts=100  x0status=blocks  SPID=on  SwTol=0  HookPort=off  NonlinearTolerance=1e-4  nMaxIteration=100  ContinueOnMaxIteration=off  RestoreLinks=warning  ResistiveCurrentMeasurement=off  Frange=[0:2:500]  Ylog=off  Xlog=on  ShowGrid=off  save=off  variable=ZData  structure=0  ZoomFFT=off  StartTime=0.0  cycles=1  DisplayStyle=1  fundamental=60  FreqAxis=off  MaxFrequency=1000  frequencyindicesteady=1  RmsSteady=1  display=off
  P_2DG : Outport
  Q_2DG : Outport  Port=2
  w_2DG : Outport  Port=3
  frequency_2DG : Outport  Port=4
  voltage_abc_DG2 : Outport  Port=5
  wires:
  Active and Reactive Power/2(Q_2DG) -> Display15/1, Scope19/1, Q_2DG/1, [Q_2DG]
  Voltage Loop Control 2 DG/1(i_s_ref_dq0_2DG) -> [i_s_ref_dq0_2DG]
  Active and Reactive Power/1(P_2DG) -> P_2DG/1, Scope18/1, Display16/1, [P_2DG]
  [P_2DG] -> Droop Control Subsystem 2 DG/2(P_2DG)
  Current Loop Control 2 DG/1(v_s_ref_dq0_2DG) -> [v_s_ref_dq0_2DG]
  Constant4/1 -> Current Loop Control 2 DG/3(w_base_2DG)
  v_dq0_2DG/1 -> Voltage Loop Control 2 DG/2(v_dq0_2DG)
  Droop Control Subsystem 2 DG/3(v_ref_dq0_2DG) -> [v_ref_dq0_2DG]
  [Q_2DG] -> Droop Control Subsystem 2 DG/1(Q_2DG)
  Droop Control Subsystem 2 DG/1(w_2DG) -> Display9/1, w_2DG/1
  i_dq0_2DG/1 -> Voltage Loop Control 2 DG/3(i_dq0_2DG)
  i_s_dq0_2DG/1 -> Current Loop Control 2 DG/2(i_s_dq0_2DG)
  Constant3/1 -> Voltage Loop Control 2 DG/4(w_base_2DG)
  [i_s_ref_dq0_2DG] -> Current Loop Control 2 DG/1(i_s_ref_dq0_2DG)
  convertion block dq to abc frame 2 DG/1(voltage_abc_DG2) -> voltage_abc_DG2/1
  [v_s_ref_dq0_2DG] -> convertion block dq to abc frame 2 DG/1(v_s_ref_dq0_2DG)
  alpha_2DG/1 -> convertion block dq to abc frame 2 DG/2(alpha_2DG)
  V_n_2DG/1 -> Droop Control Subsystem 2 DG/4(V_n_2DG)
  v_od_2DG/1 -> Active and Reactive Power/1(v_od_2DG)
  i_oq_2DG/1 -> Active and Reactive Power/4(i_oq_2DG)
  v_oq_2DG/1 -> Active and Reactive Power/3(v_oq_2DG)
  i_od_2DG/1 -> Active and Reactive Power/2(i_od_2DG)
  w_n_2DG/1 -> Droop Control Subsystem 2 DG/3(w_n_2DG)
  Droop Control Subsystem 2 DG/2(frequency_2DG) -> Display1/1, frequency_2DG/1
  [v_ref_dq0_2DG] -> Voltage Loop Control 2 DG/1(v_ref_dq0_2DG)

== system Grid_Forming_Converters_Microgrid_Github/DG 2 VCVSI/RL OUTPUT CONNECTOR 2 DG ==
  Series RLC Branch : powerlib/Elements/Series RLC Branch  LConnTagsString=__new0  RConnTagsString=__new0  BranchType=RL  Resistance=R_ci_2DG  Inductance=L_ci_2DG  SetiL0=off  InitialCurrent=0  Capacitance=1e-6  Setx0=off  InitialVoltage=0  Measurements=None
  Series RLC Branch1 : powerlib/Elements/Series RLC Branch  LConnTagsString=__new0  RConnTagsString=__new0  BranchType=RL  Resistance=R_ci_2DG  Inductance=L_ci_2DG  SetiL0=off  InitialCurrent=0  Capacitance=1e-6  Setx0=off  InitialVoltage=0  Measurements=None
  Series RLC Branch2 : powerlib/Elements/Series RLC Branch  LConnTagsString=__new0  RConnTagsString=__new0  BranchType=RL  Resistance=R_ci_2DG  Inductance=L_ci_2DG  SetiL0=off  InitialCurrent=0  Capacitance=1e-6  Setx0=off  InitialVoltage=0  Measurements=None
  Series RLC Branch3 : PMIOPort  Side=Right
  Series RLC Branch4 : PMIOPort  Port=2  Side=Left
  Series RLC Branch5 : PMIOPort  Port=3  Side=Right
  Series RLC Branch6 : PMIOPort  Port=4  Side=Left
  Series RLC Branch7 : PMIOPort  Port=5  Side=Left
  Series RLC Branch8 : PMIOPort  Port=6  Side=Right
  connections:
  Series RLC Branch1/LConn1 -- Series RLC Branch6/RConn1
  Series RLC Branch2/RConn1 -- Series RLC Branch8/RConn1
  Series RLC Branch/RConn1 -- Series RLC Branch3/RConn1
  Series RLC Branch2/LConn1 -- Series RLC Branch7/RConn1
  Series RLC Branch/LConn1 -- Series RLC Branch4/RConn1
  Series RLC Branch1/RConn1 -- Series RLC Branch5/RConn1

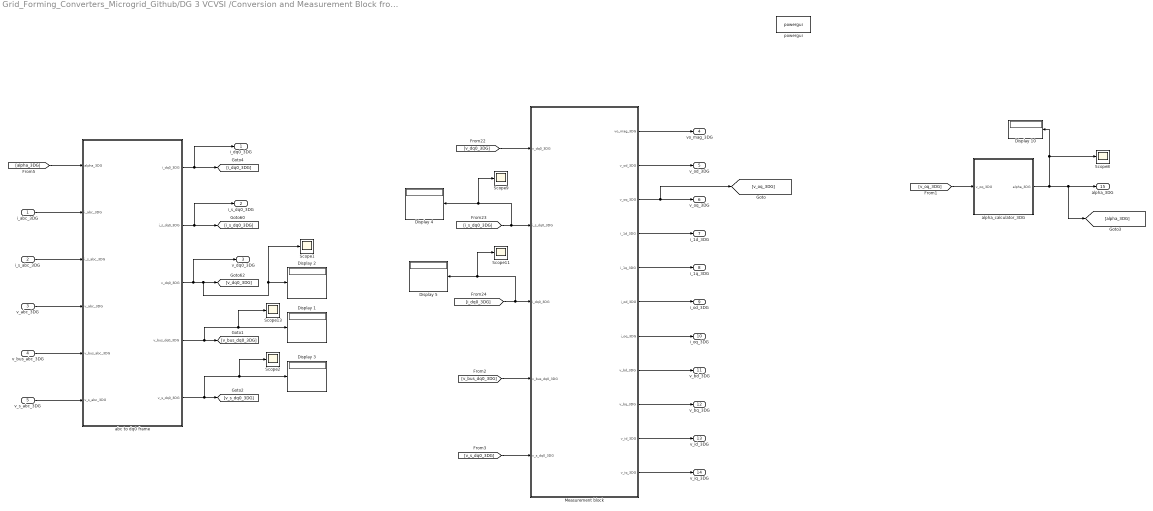
== system Grid_Forming_Converters_Microgrid_Github/DG 3 VCVSI /Conversion and Measurement Block from abc to dq0 frame ==
  i_abc_3DG : Inport
  i_s_abc_3DG : Inport  Port=2
  v_abc_3DG : Inport  Port=3
  v_bus_abc_3DG : Inport  Port=4
  v_s_abc_3DG : Inport  Port=5
  Display {1..5,10} (6 alike) : Display
      settings: Format=bank
  Measurement block : Subsystem
  Scope{1..2,8..9,11,13} (6 alike) : Scope
  abc to dq0 frame : Subsystem
  alpha_calculator_3DG : Subsystem
  powergui : powerlib/powergui  Priority=1  SimulationMode=Discrete  SampleTime=2e-6  frequency=60  Iterations=50  frequencyindice=0  Pbase=100e6  ErrMax=1e-4  UnitsV=kV  UnitsW=MW  buscounter=0  FunctionMessages=off  echomessages=off  EnableUseOfTLC=off  CurrentSourceSwitches=off  DisableSnubberDevices=off  DisableRonSwitches=off  DisableVfSwitches=off  DisplayEquations=off  AutomaticDiscreteSolvers=off  SolverType=Tustin/Backward Euler (TBE)  Interpol=off  ExternalGateDelay=off  methode=off  Ts=100  x0status=blocks  SPID=on  SwTol=0  HookPort=off  NonlinearTolerance=1e-4  nMaxIteration=100  ContinueOnMaxIteration=off  RestoreLinks=warning  ResistiveCurrentMeasurement=off  Frange=[0:2:500]  Ylog=off  Xlog=on  ShowGrid=off  save=off  variable=ZData  structure=0  ZoomFFT=off  StartTime=0.0  cycles=1  DisplayStyle=1  fundamental=60  FreqAxis=off  MaxFrequency=1000  frequencyindicesteady=1  RmsSteady=1  display=off
  i_dq0_3DG : Outport
  i_s_dq0_3DG : Outport  Port=2
  v_dq0_3DG : Outport  Port=3
  vo_mag_3DG : Outport  Port=4
  v_od_3DG : Outport  Port=5
  v_oq_3DG : Outport  Port=6
  i_1d_3DG : Outport  Port=7
  i_1q_3DG : Outport  Port=8
  i_od_3DG : Outport  Port=9
  i_oq_3DG : Outport  Port=10
  v_bd_3DG : Outport  Port=11
  v_bq_3DG : Outport  Port=12
  v_id_3DG : Outport  Port=13
  v_iq_3DG : Outport  Port=14
  alpha_3DG : Outport  Port=15
  wires:
  Measurement block/5(i_1q_3DG) -> i_1q_3DG/1
  [i_dq0_3DG] -> Scope11/1, Display 5/1, Measurement block/3(i_dq0_3DG)
  abc to dq0 frame/2(i_s_dq0_3DG) -> i_s_dq0_3DG/1, [i_s_dq0_3DG]
  i_s_abc_3DG/1 -> abc to dq0 frame/3(i_s_abc_3DG)
  abc to dq0 frame/1(i_dq0_3DG) -> i_dq0_3DG/1, [i_dq0_3DG]
  Measurement block/4(i_1d_3DG) -> i_1d_3DG/1
  Measurement block/6(i_od_3DG) -> i_od_3DG/1
  abc to dq0 frame/3(v_dq0_3DG) -> v_dq0_3DG/1, Scope1/1, Display 2/1, [v_dq0_3DG]
  [v_dq0_3DG] -> Measurement block/1(v_dq0_3DG)
  i_abc_3DG/1 -> abc to dq0 frame/2(i_abc_3DG)
  Measurement block/2(v_od_3DG) -> v_od_3DG/1
  Measurement block/3(v_oq_3DG) -> [v_oq_3DG], v_oq_3DG/1
  v_abc_3DG/1 -> abc to dq0 frame/4(v_abc_3DG)
  Measurement block/7(i_oq_3DG) -> i_oq_3DG/1
  alpha_calculator_3DG/1(alpha_3DG) -> [alpha_3DG], alpha_3DG/1, Display 10/1, Scope8/1
  [v_oq_3DG] -> alpha_calculator_3DG/1(v_oq_3DG)
  [alpha_3DG] -> abc to dq0 frame/1(alpha_3DG)
  Measurement block/1(vo_mag_3DG) -> vo_mag_3DG/1
  [i_s_dq0_3DG] -> Scope9/1, Display 4/1, Measurement block/2(i_s_dq0_3DG)
  v_bus_abc_3DG/1 -> abc to dq0 frame/5(v_bus_abc_3DG)
  v_s_abc_3DG/1 -> abc to dq0 frame/6(v_s_abc_3DG)
  abc to dq0 frame/4(v_bus_dq0_3DG) -> Scope13/1, Display 1/1, [v_bus_dq0_3DG]
  abc to dq0 frame/5(v_s_dq0_3DG) -> Scope2/1, Display 3/1, [v_s_dq0_3DG]
  [v_bus_dq0_3DG] -> Measurement block/4(v_bus_dq0_3DG)
  [v_s_dq0_3DG] -> Measurement block/5(v_s_dq0_3DG)
  Measurement block/8(v_bd_3DG) -> v_bd_3DG/1
  Measurement block/9(v_bq_3DG) -> v_bq_3DG/1
  Measurement block/10(v_id_3DG) -> v_id_3DG/1
  Measurement block/11(v_iq_3DG) -> v_iq_3DG/1

== system Grid_Forming_Converters_Microgrid_Github/DG 3 VCVSI /LC FILTER 3 DG ==
  C_a : powerlib/Elements/Series RLC Branch  LConnTagsString=__new0  RConnTagsString=__new0  BranchType=C  Resistance=1  Inductance=1e-3  SetiL0=off  InitialCurrent=0  Capacitance=C_fi_3DG  Setx0=off  InitialVoltage=165  Measurements=None
  C_b : powerlib/Elements/Series RLC Branch  LConnTagsString=__new0  RConnTagsString=__new0  BranchType=C  Resistance=1  Inductance=1e-3  SetiL0=off  InitialCurrent=0  Capacitance=C_fi_3DG  Setx0=off  InitialVoltage=165  Measurements=None
  C_c1 : powerlib/Elements/Series RLC Branch  LConnTagsString=__new0  RConnTagsString=__new0  BranchType=C  Resistance=1  Inductance=1e-3  SetiL0=off  InitialCurrent=0  Capacitance=C_fi_3DG  Setx0=off  InitialVoltage=165  Measurements=None
  Ground2 : powerlib/Elements/Ground  LConnTagsString=a
  Series RLC Branch : powerlib/Elements/Series RLC Branch  LConnTagsString=__new0  RConnTagsString=__new0  BranchType=L  Resistance=1  Inductance=L_fi_3DG  SetiL0=off  InitialCurrent=0  Capacitance=1e-6  Setx0=off  InitialVoltage=0  Measurements=None
  Series RLC Branch1 : powerlib/Elements/Series RLC Branch  LConnTagsString=__new0  RConnTagsString=__new0  BranchType=R  Resistance=R_fi_3DG  Inductance=L_i_1DG  SetiL0=off  InitialCurrent=0  Capacitance=1e-6  Setx0=off  InitialVoltage=0  Measurements=None
  Series RLC Branch2 : powerlib/Elements/Series RLC Branch  LConnTagsString=__new0  RConnTagsString=__new0  BranchType=R  Resistance=R_fi_3DG  Inductance=L_i_1DG  SetiL0=off  InitialCurrent=0  Capacitance=1e-6  Setx0=off  InitialVoltage=0  Measurements=None
  Series RLC Branch3 : powerlib/Elements/Series RLC Branch  LConnTagsString=__new0  RConnTagsString=__new0  BranchType=L  Resistance=1  Inductance=L_fi_3DG  SetiL0=off  InitialCurrent=0  Capacitance=1e-6  Setx0=off  InitialVoltage=0  Measurements=None
  Series RLC Branch4 : powerlib/Elements/Series RLC Branch  LConnTagsString=__new0  RConnTagsString=__new0  BranchType=R  Resistance=R_fi_3DG  Inductance=R_fi_1DG  SetiL0=off  InitialCurrent=0  Capacitance=1e-6  Setx0=off  InitialVoltage=0  Measurements=None
  Series RLC Branch5 : powerlib/Elements/Series RLC Branch  LConnTagsString=__new0  RConnTagsString=__new0  BranchType=L  Resistance=1  Inductance=L_fi_3DG  SetiL0=off  InitialCurrent=0  Capacitance=1e-6  Setx0=off  InitialVoltage=0  Measurements=None
  Series RLC Branch6 : PMIOPort  Side=Left
  Series RLC Branch7 : PMIOPort  Port=2  Side=Right
  Series RLC Branch8 : PMIOPort  Port=3  Side=Left
  Series RLC Branch9 : PMIOPort  Port=4  Side=Right
  Series RLC Branch10 : PMIOPort  Port=5  Side=Left
  Series RLC Branch11 : PMIOPort  Port=6  Side=Right
  connections:
  Series RLC Branch7/RConn1 -- C_c1/LConn1 -- Series RLC Branch/RConn1
  Series RLC Branch8/RConn1 -- Series RLC Branch2/LConn1
  Series RLC Branch6/RConn1 -- Series RLC Branch1/LConn1
  Series RLC Branch9/RConn1 -- C_b/LConn1 -- Series RLC Branch3/RConn1
  Series RLC Branch11/RConn1 -- C_a/LConn1 -- Series RLC Branch5/RConn1
  Series RLC Branch10/RConn1 -- Series RLC Branch4/LConn1
  C_b/RConn1 -- C_c1/RConn1 -- Ground2/LConn1 -- C_a/RConn1
  Series RLC Branch/LConn1 -- Series RLC Branch1/RConn1
  Series RLC Branch3/LConn1 -- Series RLC Branch2/RConn1
  Series RLC Branch4/RConn1 -- Series RLC Branch5/LConn1

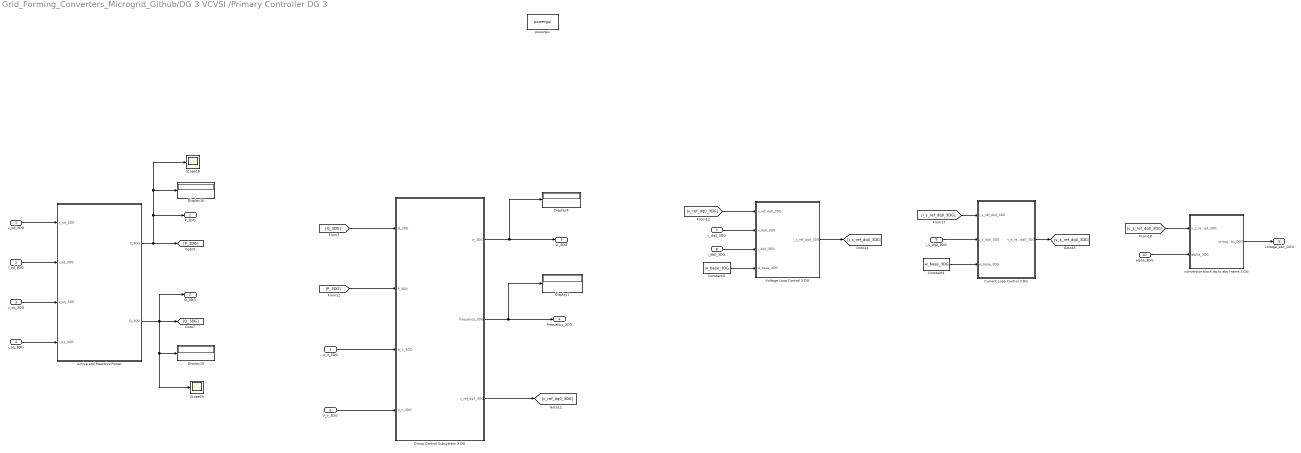
== system Grid_Forming_Converters_Microgrid_Github/DG 3 VCVSI /Primary Controller DG 3 ==
  v_od_3DG : Inport
  i_od_3DG : Inport  Port=2
  v_oq_3DG : Inport  Port=3
  i_oq_3DG : Inport  Port=4
  w_n_3DG : Inport  Port=5
  V_n_3DG : Inport  Port=6
  v_dq0_3DG : Inport  Port=7
  i_dq0_3DG : Inport  Port=8
  i_s_dq0_3DG : Inport  Port=9
  alpha_3DG : Inport  Port=10
  Active and Reactive Power : Subsystem
  Constant3 : Constant  Value=w_base_3DG
  Constant4 : Constant  Value=w_base_3DG
  Current Loop Control 3 DG : Subsystem
  Display{1,9,15..16} (4 alike) : Display
  Droop Control Subsystem 3 DG : Subsystem
  Scope18 : Scope
  Scope19 : Scope
  Voltage Loop Control 3 DG : Subsystem
  convertion block dq to abc frame 3 DG : Subsystem
  powergui : powerlib/powergui  Priority=1  SimulationMode=Discrete  SampleTime=Ts_1DG  frequency=60  Iterations=50  frequencyindice=0  Pbase=100e6  ErrMax=1e-4  UnitsV=kV  UnitsW=MW  buscounter=0  FunctionMessages=off  echomessages=off  EnableUseOfTLC=off  CurrentSourceSwitches=off  DisableSnubberDevices=off  DisableRonSwitches=off  DisableVfSwitches=off  DisplayEquations=off  AutomaticDiscreteSolvers=off  SolverType=Tustin/Backward Euler (TBE)  Interpol=off  ExternalGateDelay=off  methode=off  Ts=100  x0status=blocks  SPID=on  SwTol=0  HookPort=off  NonlinearTolerance=1e-4  nMaxIteration=100  ContinueOnMaxIteration=off  RestoreLinks=warning  ResistiveCurrentMeasurement=off  Frange=[0:2:500]  Ylog=off  Xlog=on  ShowGrid=off  save=off  variable=ZData  structure=0  ZoomFFT=off  StartTime=0.0  cycles=1  DisplayStyle=1  fundamental=60  FreqAxis=off  MaxFrequency=1000  frequencyindicesteady=1  RmsSteady=1  display=off
  P_3DG : Outport
  Q_3DG : Outport  Port=2
  w_3DG : Outport  Port=3
  frequency_3DG : Outport  Port=4
  voltage_abc_DG3 : Outport  Port=5
  wires:
  Active and Reactive Power/2(Q_3DG) -> Display15/1, Scope19/1, Q_3DG/1, [Q_3DG]
  Voltage Loop Control 3 DG/1(i_s_ref_dq0_3DG) -> [i_s_ref_dq0_3DG]
  Active and Reactive Power/1(P_3DG) -> P_3DG/1, Scope18/1, Display16/1, [P_3DG]
  [v_ref_dq0_3DG] -> Voltage Loop Control 3 DG/1(v_ref_dq0_3DG)
  [P_3DG] -> Droop Control Subsystem 3 DG/2(P_3DG)
  Current Loop Control 3 DG/1(v_s_ref_dq0_3DG) -> [v_s_ref_dq0_3DG]
  Constant4/1 -> Current Loop Control 3 DG/3(w_base_3DG)
  v_dq0_3DG/1 -> Voltage Loop Control 3 DG/2(v_dq0_3DG)
  Droop Control Subsystem 3 DG/3(v_ref_dq0_3DG) -> [v_ref_dq0_3DG]
  [Q_3DG] -> Droop Control Subsystem 3 DG/1(Q_3DG)
  Droop Control Subsystem 3 DG/1(w_3DG) -> Display9/1, w_3DG/1
  i_dq0_3DG/1 -> Voltage Loop Control 3 DG/3(i_dq0_3DG)
  i_s_dq0_3DG/1 -> Current Loop Control 3 DG/2(i_s_dq0_3DG)
  Constant3/1 -> Voltage Loop Control 3 DG/4(w_base_3DG)
  [i_s_ref_dq0_3DG] -> Current Loop Control 3 DG/1(i_s_ref_dq0_3DG)
  convertion block dq to abc frame 3 DG/1(voltage_abc_DG3) -> voltage_abc_DG3/1
  [v_s_ref_dq0_3DG] -> convertion block dq to abc frame 3 DG/1(v_s_ref_dq0_3DG)
  alpha_3DG/1 -> convertion block dq to abc frame 3 DG/2(alpha_3DG)
  V_n_3DG/1 -> Droop Control Subsystem 3 DG/4(V_n_3DG)
  v_od_3DG/1 -> Active and Reactive Power/1(v_od_3DG)
  i_oq_3DG/1 -> Active and Reactive Power/4(i_oq_3DG)
  v_oq_3DG/1 -> Active and Reactive Power/3(v_oq_3DG)
  i_od_3DG/1 -> Active and Reactive Power/2(i_od_3DG)
  w_n_3DG/1 -> Droop Control Subsystem 3 DG/3(w_n_3DG)
  Droop Control Subsystem 3 DG/2(frequency_3DG) -> Display1/1, frequency_3DG/1
